simulink model "ACFTSim"  (R2024b)
settings: Solver=ode4  StartTime=0.0  StopTime=inf  FixedStep=0.01  RelTol=1e-3  EnableMultiTasking=on
undefined symbols (not defined in the file): Earth, Inertia, Receive, Send, Trimming, WGS84
libraries: aerolibfltsims x2, Aerodynamics x1, Atmospheric x1, EqM x1, vrlib x1, Propulsion x1, aerolibtransform2 x1, aerolibanim x1
settings Model: Creator=ada09  LastModifiedBy=ada09
settings DataIOCC: ExternalInput=getinputstruct(opreport)  InitialState=getstatestruct(opreport)  LoadExternalInput=on  LoadInitialState=on  SaveState=on  ReturnWorkspaceOutputs=off
settings DebuggingCC: InheritedTsInSrcMsg=none
settings ModelReferenceCC: EnableRefExpFcnMdlSchedulingChecks=on

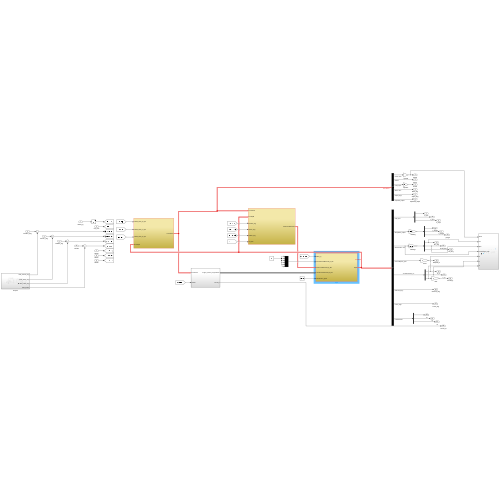
[thumbnail: Simulink's stored preview of the top-level diagram]
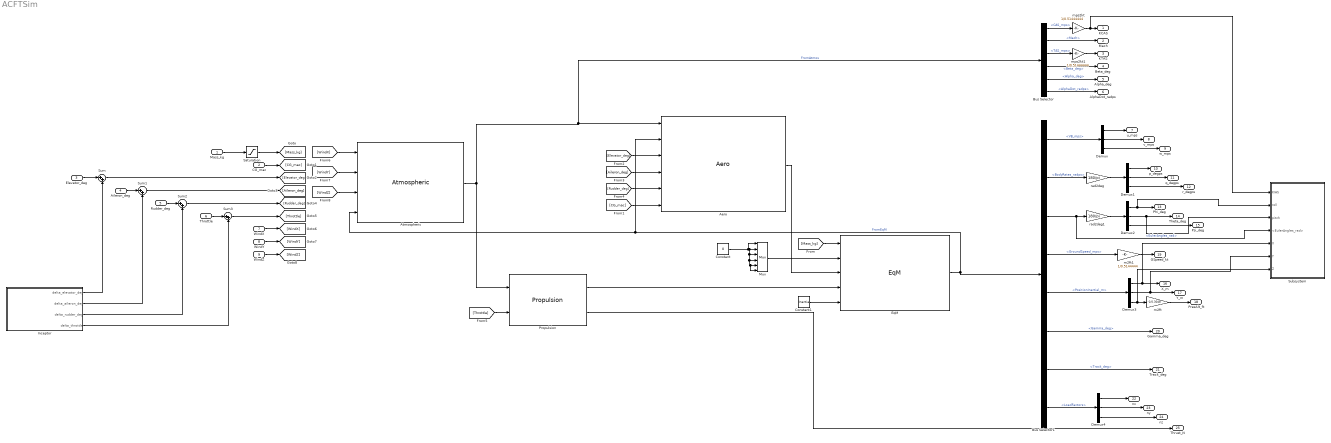
== system ACFTSim ==
  Mass_kg : Inport
  CG_mac : Inport  Port=2
  Elevator_deg : Inport  Port=3
  Aileron_deg : Inport  Port=4
  Rudder_deg : Inport  Port=5
  Throttle : Inport  Port=6
  WindX : Inport  Port=7
  WindY : Inport  Port=8
  WindZ : Inport  Port=9
  Aero : Aerodynamics/Aero  SystemSampleTime=-1  VariantActivationTime=update diagram  AllowFlexibleInterface=on  Latency=0  AutoFrameSizeCalculation=off
  Atmospheric : Atmospheric/Atmospheric  SystemSampleTime=-1  VariantActivationTime=update diagram  AllowFlexibleInterface=on  Latency=0  AutoFrameSizeCalculation=off
  Bus Selector : BusSelector  OutputSignals=CAS_mps,Mach,TAS_mps,Beta_deg,Alpha_deg,AlphaDot_radps
  Bus Selector1 : BusSelector  OutputSignals=VB_mps,BodyRates_radps,EulerAngles_rad,GroundSpeed_mps,PositionInertial_m,Gamma_deg,Track_deg,LoadFactors
  Constant : Constant  Value=0
  Constant1 : Constant  Value=Inertia
  Demux{,1..4} (5 alike) : Demux  Outputs=3
  EqM : EqM/EqM  SystemSampleTime=-1  VariantActivationTime=update diagram  AllowFlexibleInterface=on  Latency=0  AutoFrameSizeCalculation=off
  Inceptor : Subsystem
  Mux : Mux  Inputs=6
  Propulsion : Propulsion/Propulsion  SystemSampleTime=-1  VariantActivationTime=update diagram  AllowFlexibleInterface=on  Latency=0  AutoFrameSizeCalculation=off
  Saturation : Saturate  UpperLimit=inf  LowerLimit=0.1
  Subsystem : Subsystem
  Sum{,1..3} (4 alike) : Sum  Inputs=|++
  m2ft : Gain  Gain=-1/0.3048
  m2ft1 : Gain  Gain=1/0.5144444
  mps2kt : Gain  Gain=1/0.51444444
  mps2kt1 : Gain  Gain=1/0.51444444
  rad2deg : Gain  Gain=180/pi
  rad2deg1 : Gain  Gain=180/pi
  KCAS : Outport
  Mach : Outport  Port=2
  KTAS : Outport  Port=3
  Beta_deg : Outport  Port=4
  "Alpha_deg " : Outport  Port=5
  AlphaDot_radps : Outport  Port=6
  u_mps : Outport  Port=7
  v_mps : Outport  Port=8
  w_mps : Outport  Port=9
  p_degps : Outport  Port=10
  q_degps : Outport  Port=11
  r_degps : Outport  Port=12
  Phi_deg : Outport  Port=13
  Theta_deg : Outport  Port=14
  Psi_deg : Outport  Port=15
  X_m : Outport  Port=16
  Y_m : Outport  Port=17
  PresAlt_ft : Outport  Port=18
  GSpeed_kt : Outport  Port=19
  Gamma_deg : Outport  Port=20
  Track_deg : Outport  Port=21
  nx : Outport  Port=22
  ny : Outport  Port=23
  nz : Outport  Port=24
  Thrust_N : Outport  Port=25
  wires:
  Atmospheric/1 -> Propulsion/1, Bus Selector/1, Aero/1  "FromAtmos"
  Propulsion/1 -> EqM/4
  EqM/1 -> Bus Selector1/1, Atmospheric/4, Aero/2  "FromEqM"
  Constant/1 -> Mux/1, Mux/2, Mux/6, Mux/5, Mux/4, Mux/3
  Mass_kg/1 -> Saturation/1
  CG_mac/1 -> [CG_mac]
  WindX/1 -> [WindX]
  WindY/1 -> [WindY]
  WindZ/1 -> [WindZ]
  [WindX] -> Atmospheric/1
  [WindY] -> Atmospheric/2
  [WindZ] -> Atmospheric/3
  [Throttle] -> Propulsion/2
  Constant1/1 -> EqM/5
  [CG_mac] -> Aero/6
  [Elevator_deg] -> Aero/3
  [Aileron_deg] -> Aero/4
  [Rudder_deg] -> Aero/5
  Propulsion/2 -> Thrust_N/1
  Bus Selector/1 -> mps2kt/1  "<CAS_mps>"
  Bus Selector/2 -> Mach/1  "<Mach>"
  mps2kt/1 -> Subsystem/1(KIAS), KCAS/1
  Bus Selector/3 -> mps2kt1/1  "<TAS_mps>"
  mps2kt1/1 -> KTAS/1
  Bus Selector/4 -> Beta_deg/1  "<Beta_deg>"
  Bus Selector/5 -> "Alpha_deg "/1  "<Alpha_deg>"
  Bus Selector/6 -> AlphaDot_radps/1  "<AlphaDot_radps>"
  Bus Selector1/1 -> Demux/1  "<VB_mps>"
  Demux/1 -> u_mps/1
  Demux/2 -> v_mps/1
  Demux/3 -> w_mps/1
  Bus Selector1/2 -> rad2deg/1  "<BodyRates_radps>"
  rad2deg/1 -> Demux1/1
  Demux1/1 -> p_degps/1
  Demux1/2 -> q_degps/1
  Demux1/3 -> r_degps/1
  Bus Selector1/3 -> Subsystem/4(<EulerAngles_rad>), rad2deg1/1  "<EulerAngles_rad>"
  rad2deg1/1 -> Demux2/1
  Demux2/1 -> Subsystem/2(roll), Phi_deg/1
  Demux2/2 -> Subsystem/3(pitch), Theta_deg/1
  Demux2/3 -> Psi_deg/1
  Bus Selector1/5 -> Demux3/1  "<PositionInertial_m>"
  Demux3/1 -> Subsystem/5(X), X_m/1
  Demux3/2 -> Y_m/1, Subsystem/6(Y)
  Demux3/3 -> Subsystem/7(Z), m2ft/1
  m2ft/1 -> PresAlt_ft/1
  Bus Selector1/4 -> m2ft1/1  "<GroundSpeed_mps>"
  m2ft1/1 -> GSpeed_kt/1
  Bus Selector1/6 -> Gamma_deg/1  "<Gamma_deg>"
  Bus Selector1/7 -> Track_deg/1  "<Track_deg>"
  Bus Selector1/8 -> Demux4/1  "<LoadFactors>"
  Demux4/3 -> nz/1
  Demux4/1 -> nx/1
  Demux4/2 -> ny/1
  Aero/1 -> EqM/3
  Mux/1 -> EqM/2
  [Mass_kg] -> EqM/1
  Saturation/1 -> [Mass_kg]
  Inceptor/3(delta_rudder_deg) -> Sum2/2
  Inceptor/2(delta_aileron_deg) -> Sum1/2
  Inceptor/1(delta_elevator_deg) -> Sum/2
  Inceptor/4(delta_throttle) -> Sum3/2
  Elevator_deg/1 -> Sum/1
  Sum/1 -> [Elevator_deg]
  Aileron_deg/1 -> Sum1/1
  Sum1/1 -> [Aileron_deg]
  Rudder_deg/1 -> Sum2/1
  Sum2/1 -> [Rudder_deg]
  Throttle/1 -> Sum3/1
  Sum3/1 -> [Throttle]

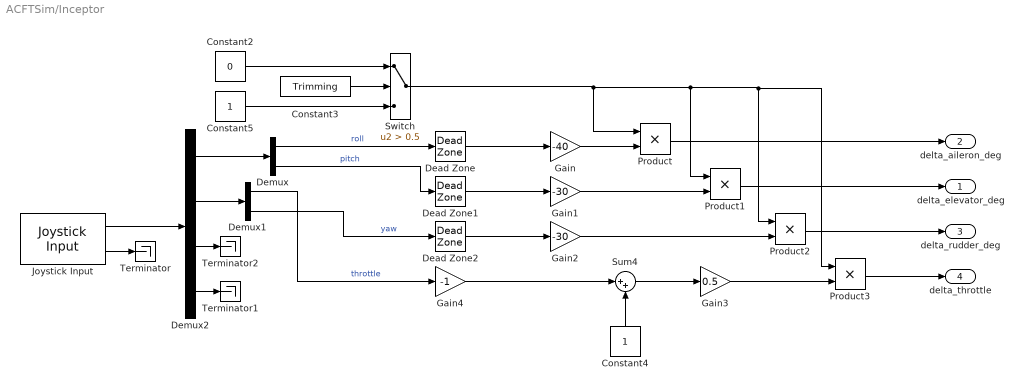
== system ACFTSim/Inceptor ==
  Constant2 : Constant  Value=0
  Constant3 : Constant  Value=Trimming
  Constant4 : Constant
  Constant5 : Constant
  Dead Zone : DeadZone  LowerValue=-0.05  UpperValue=0.05
  Dead Zone1 : DeadZone  LowerValue=-0.05  UpperValue=0.05
  Dead Zone2 : DeadZone  LowerValue=-0.05  UpperValue=0.05
  Demux : Demux  Outputs=2
  Demux1 : Demux  Outputs=2
  Demux2 : Demux
  Gain : Gain  Gain=-40
  Gain1 : Gain  Gain=-30
  Gain2 : Gain  Gain=-30
  Gain3 : Gain  Gain=0.5
  Gain4 : Gain  Gain=-1
  Joystick Input : vrlib/Joystick Input  joyid=1  adjustports=on  forcefeed=off
  Product{,1..3} (4 alike) : Product
  Sum4 : Sum  Inputs=|++
  Switch : Switch  Criteria=u2 > Threshold  Threshold=0.5  SaturateOnIntegerOverflow=off  InputSameDT=off
  Terminator : Terminator
  Terminator1 : Terminator
  Terminator2 : Terminator
  delta_elevator_deg : Outport
  delta_aileron_deg : Outport  Port=2
  delta_rudder_deg : Outport  Port=3
  delta_throttle : Outport  Port=4
  wires:
  Switch/1 -> Product/1, Product2/1, Product3/1, Product1/1
  Constant3/1 -> Switch/2
  Product2/1 -> delta_rudder_deg/1
  Dead Zone2/1 -> Gain2/1
  Sum4/1 -> Gain3/1
  Constant5/1 -> Switch/3
  Product/1 -> delta_aileron_deg/1
  Dead Zone/1 -> Gain/1
  Gain/1 -> Product/2
  Constant2/1 -> Switch/1
  Gain3/1 -> Product3/2
  Gain4/1 -> Sum4/1
  Dead Zone1/1 -> Gain1/1
  Gain2/1 -> Product2/2
  Gain1/1 -> Product1/2
  Constant4/1 -> Sum4/2
  Product1/1 -> delta_elevator_deg/1
  Product3/1 -> delta_throttle/1
  Demux1/2 -> Dead Zone2/1  "yaw"
  Demux1/1 -> Gain4/1  "throttle"
  Demux/2 -> Dead Zone1/1  "pitch"
  Demux/1 -> Dead Zone/1  "roll"
  Demux2/2 -> Demux1/1
  Demux2/1 -> Demux/1
  Demux2/3 -> Terminator2/1
  Demux2/4 -> Terminator1/1
  Joystick Input/2 -> Terminator/1
  Joystick Input/1 -> Demux2/1

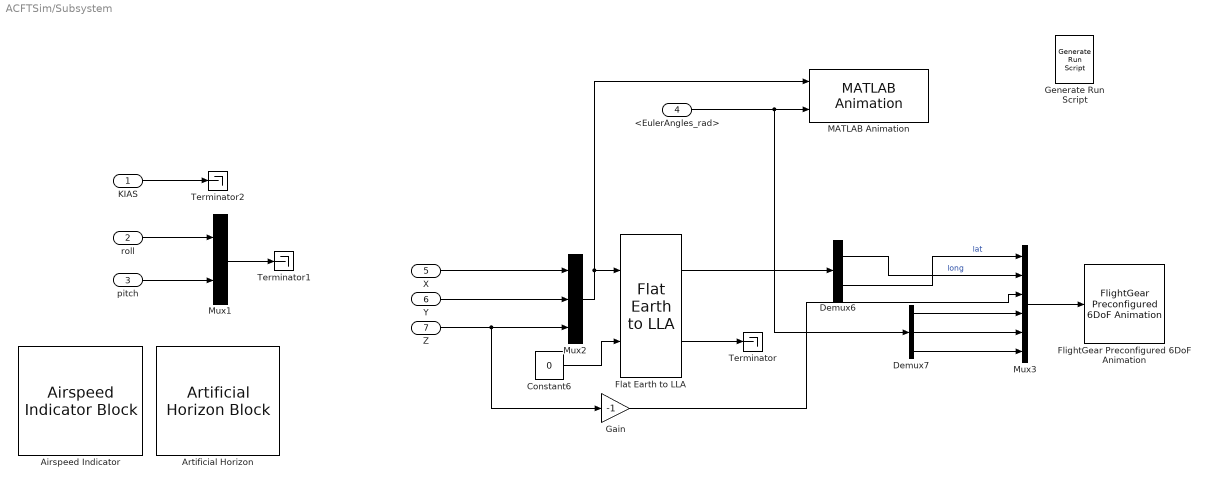
== system ACFTSim/Subsystem ==
  KIAS : Inport
  roll : Inport  Port=2
  pitch : Inport  Port=3
  <EulerAngles_rad> : Inport  Port=4
  X : Inport  Port=5
  Y : Inport  Port=6
  Z : Inport  Port=7
  Airspeed Indicator : AirspeedIndicatorBlock  ScaleMin=0
  Artificial Horizon : ArtificialHorizonBlock
  Constant6 : Constant  Value=0
  Demux6 : Demux  Outputs=2
  Demux7 : Demux  Outputs=3
  Flat Earth to LLA : aerolibtransform2/Flat Earth to LLA  units=Metric (MKS)  ptype=Earth (WGS84)  F=1/298.257223563  R=6378137  refPosPort=off  LL0=[0 10]  psi=0
  FlightGear Preconfigured 6DoF Animation : aerolibfltsims/FlightGear Preconfigured 6DoF Animation  xFlightGearVersion=v2019.1  DestinationIpAddress=127.0.0.1  DestinationPort=5502  SampleTime=0.01  packetVersion=24
  Gain : Gain  Gain=-1
  Generate Run Script : aerolibfltsims/Generate Run Script  Architecture=Win64  dataFlow=Send-Receive  GeometryModelName=c172p  AirportId=KSFO  RunwayId=10L  InitialAltitude=7224  InitialHeading=113  OffsetDistance=4.72  OffsetAzimuth=0  InstallScenery=on  DisableShaders=off  OriginAddress=127.0.0.1  DestinationPort=5502  OriginPort=5505  LocalAddress=127.0.0.1  OutputFileName=runfg.bat  FlightGearBaseDirectory=C:\Program Files\FlightGear
  MATLAB Animation : aerolibanim/MATLAB Animation  Tag=Matlab Animation 6 DOF  Vehicles=1  Geometries='astredwedge.mat'  BoundingBoxCoordinates=[-50,50,-50,50,-50,50]  CameraOffset=[-150,-50,0]  CameraViewAngle=3  SampleTime=0.01  FigurePosition=[892,242,400,289]
  Mux1 : Mux  Inputs=2
  Mux2 : Mux  Inputs=3
  Mux3 : Mux  Inputs=6
  Terminator : Terminator
  Terminator1 : Terminator
  Terminator2 : Terminator
  wires:
  KIAS/1 -> Terminator2/1
  pitch/1 -> Mux1/2
  roll/1 -> Mux1/1
  Mux1/1 -> Terminator1/1
  Flat Earth to LLA/2 -> Terminator/1
  <EulerAngles_rad>/1 -> MATLAB Animation/2, Demux7/1
  Z/1 -> Gain/1, Mux2/3
  Mux2/1 -> Flat Earth to LLA/1, MATLAB Animation/1
  Demux7/3 -> Mux3/6
  Constant6/1 -> Flat Earth to LLA/2
  Flat Earth to LLA/1 -> Demux6/1
  Demux7/1 -> Mux3/4
  Mux3/1 -> FlightGear Preconfigured 6DoF Animation/1
  Demux7/2 -> Mux3/5
  Y/1 -> Mux2/2
  X/1 -> Mux2/1
  Demux6/2 -> Mux3/1  "lat"
  Demux6/1 -> Mux3/2  "long"
  Gain/1 -> Mux3/3
